simulink model "VTOL_sim_f_no_zeros"  (R2016b)
settings: Solver=ode45  StartTime=0.0  StopTime=200  RelTol=1e-3  EnableMultiTasking=on
InitFcn:
  | addpath ./..
  | VTOL_param
  | VTOLParamHWf_longitudinal
  | VTOLParamHWf_lateral
values from neighbouring files (symbols this model uses):
  denCh = [1/0.8 1]    [VTOLParamHWf_longitudinal.m]
  denth = [1/12 1]    [VTOLParamHWf_lateral.m]
  denz = [1/1 1]    [VTOLParamHWf_lateral.m]
  Kh = 0.066    [VTOLParamHWf_longitudinal.m]
  Kth = 0.31    [VTOLParamHWf_lateral.m]
  Kz = -0.006    [VTOLParamHWf_lateral.m]
  numCh = [1/0.14 1]    [VTOLParamHWf_longitudinal.m]
  numth = [1/1.6 1]    [VTOLParamHWf_lateral.m]
  numz = [1/0.18 1]    [VTOLParamHWf_lateral.m]
undefined symbols (not defined in the file or in its folder): P, VTOL_animation
settings Model: Creator=beard  LastModifiedBy=mclain
settings DataIOCC: LimitDataPoints=on  SaveFormat=Array  SignalLoggingSaveFormat=ModelDataLogs
settings OptimizationCC: ExpressionDepthLimit=2147483647  InitFltsAndDblsToZero=on  LifeSpan=inf
settings DebuggingCC: UnderspecifiedInitializationDetection=Classic  MergeDetectMultiDrivingBlocksExec=none  SolverPrmCheckMsg=warning  FcnCallInpInsideContextMsg=warning  StateNameClashWarn=warning  SFUnexpectedBacktrackingDiag=warning  SFNoUnconditionalDefaultTransitionDiag=warning  SFExecutionAtInitializationDiag=none
settings HardwareCC: ProdBitPerPointer=32  ProdBitPerSizeT=32  ProdBitPerPtrDiffT=32  ProdLargestAtomicFloat=None  ProdIntDivRoundTo=Undefined  ProdEndianess=Unspecified  ProdWordSize=32  ProdHWDeviceType=32-bit Generic
settings ModelReferenceCC: PropagateSignalLabelsOutOfModel=off
settings GRTTargetCC: TargetLangStandard=C89/C90 (ANSI)  GeneratePreprocessorConditionals=Disable all  CombineOutputUpdateFcns=off  GRTInterface=on
settings ConfigComp: CovMetricSettings=dw  CovHtmlReporting=on  CovSaveCumulativeToWorkspaceVar=on  CovSaveSingleToWorkspaceVar=on  CovExternalEMLEnable=off

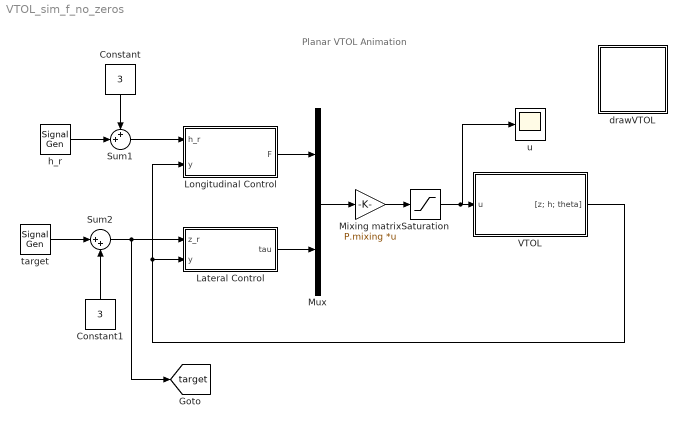
== system VTOL_sim_f_no_zeros ==
  note: Planar VTOL Animation
  Constant : Constant  Value=3
  Constant1 : Constant  Value=3
  Lateral Control : Subsystem
  Longitudinal Control : Subsystem
  Mixing matrix : Gain  Gain=P.mixing  Multiplication=Matrix(K*u)
  Mux : Mux  Inputs=2
  Saturation : Saturate  UpperLimit=100  LowerLimit=0
  Sum1 : Sum  Inputs=++|
  Sum2 : Sum  Inputs=|++
  VTOL : Subsystem
  drawVTOL : Subsystem
      mask Display: image(imread('tv.jpg'))
  h_r : SignalGenerator  WaveForm=square  Amplitude=2.5  Frequency=.01
  target : SignalGenerator  WaveForm=square  Amplitude=2  Frequency=.015
  u : Scope
  tag scope: target=global
  wires:
  VTOL/1("[z; h; theta]") -> Longitudinal Control/2(y), Lateral Control/2(y)
  Mux/1 -> Mixing matrix/1
  Mixing matrix/1 -> Saturation/1
  Longitudinal Control/1(F) -> Mux/1
  Lateral Control/1(tau) -> Mux/2
  Constant/1 -> Sum1/1
  Sum1/1 -> Longitudinal Control/1(h_r)
  h_r/1 -> Sum1/2
  target/1 -> Sum2/1
  Constant1/1 -> Sum2/2
  Saturation/1 -> u/1, VTOL/1(u)
  Sum2/1 -> [target], Lateral Control/1(z_r)

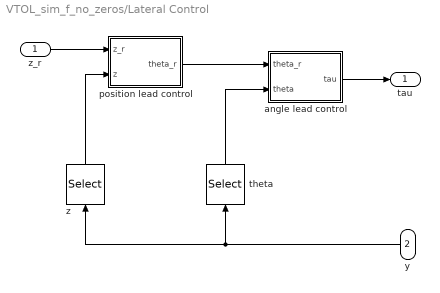
== system VTOL_sim_f_no_zeros/Lateral Control ==
  z_r : Inport
  y : Inport  Port=2
  "angle lead control " : Subsystem
  position lead control : Subsystem
  theta : Selector  InputPortWidth=3  IndexOptions=Index vector (dialog)  Indices=[3]  OutputSizes=1
  z : Selector  InputPortWidth=3  IndexOptions=Index vector (dialog)  Indices=[1]  OutputSizes=1
  tau : Outport
  wires:
  y/1 -> z/1, theta/1
  position lead control/1(theta_r) -> "angle lead control "/1(theta_r)
  theta/1 -> "angle lead control "/2(theta)
  z_r/1 -> position lead control/1(z_r)
  z/1 -> position lead control/2(z)
  "angle lead control "/1(tau) -> tau/1

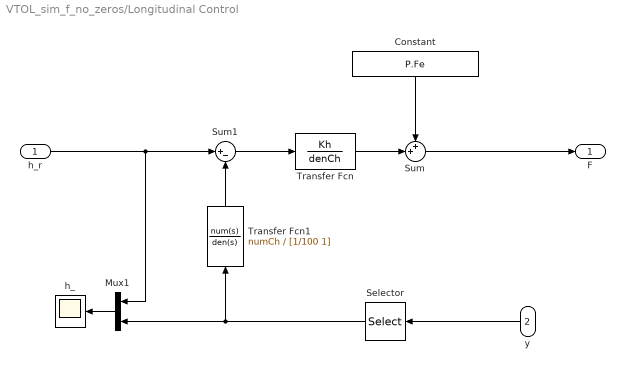
== system VTOL_sim_f_no_zeros/Longitudinal Control ==
  h_r : Inport
  y : Inport  Port=2
  Constant : Constant  Value=P.Fe
  Mux1 : Mux  Inputs=2
  Selector : Selector  InputPortWidth=3  IndexOptions=Index vector (dialog)  Indices=[2]  OutputSizes=1
  Sum : Sum  Inputs=++|
  Sum1 : Sum  Inputs=|+-
  Transfer Fcn : TransferFcn  Numerator=Kh  Denominator=denCh
  Transfer Fcn1 : TransferFcn  Numerator=numCh  Denominator=[1/100 1]
  h_ : Scope
  F : Outport
  wires:
  Selector/1 -> Transfer Fcn1/1, Mux1/2
  Sum/1 -> F/1
  Mux1/1 -> h_/1
  Constant/1 -> Sum/1
  h_r/1 -> Sum1/1, Mux1/1
  Sum1/1 -> Transfer Fcn/1
  y/1 -> Selector/1
  Transfer Fcn/1 -> Sum/2
  Transfer Fcn1/1 -> Sum1/2

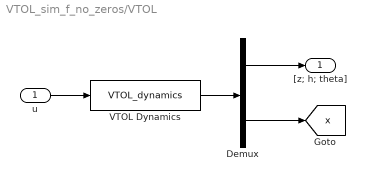
== system VTOL_sim_f_no_zeros/VTOL ==
  u : Inport
  Demux : Demux  Outputs=[3;6]
  VTOL Dynamics : S-Function  FunctionName=VTOL_dynamics  Parameters=P  SFunctionDeploymentMode=off  EnableBusSupport=off
  "[z; h; theta]" : Outport
  tag scope: x=global
  wires:
  u/1 -> VTOL Dynamics/1
  VTOL Dynamics/1 -> Demux/1
  Demux/1 -> "[z; h; theta]"/1
  Demux/2 -> [x]

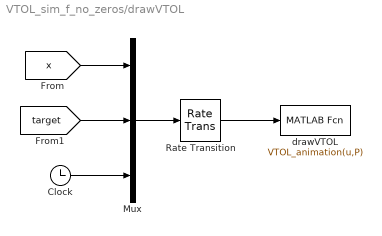
== system VTOL_sim_f_no_zeros/drawVTOL ==
  Clock : Clock
  Mux : Mux  Inputs=3
  Rate Transition : RateTransition  OutPortSampleTime=P.t_plot
  drawVTOL : MATLABFcn  MATLABFcn=VTOL_animation(u,P)  OutputDimensions=0
  wires:
  Mux/1 -> Rate Transition/1
  [x] -> Mux/1
  Clock/1 -> Mux/3
  Rate Transition/1 -> drawVTOL/1
  [target] -> Mux/2

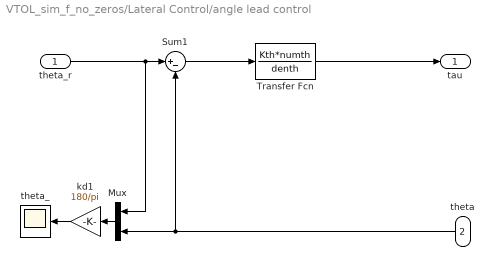
== system VTOL_sim_f_no_zeros/Lateral Control/angle lead control  ==
  theta_r : Inport
  theta : Inport  Port=2
  Mux : Mux  Inputs=2
  Sum1 : Sum  Inputs=|+-
  Transfer Fcn : TransferFcn  Numerator=Kth*numth  Denominator=denth
  kd1 : Gain  Gain=180/pi
  theta_ : Scope
  tau : Outport
  wires:
  theta_r/1 -> Sum1/1, Mux/1
  theta/1 -> Sum1/2, Mux/2
  Sum1/1 -> Transfer Fcn/1
  kd1/1 -> theta_/1
  Mux/1 -> kd1/1
  Transfer Fcn/1 -> tau/1

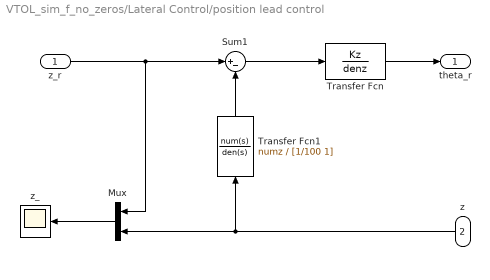
== system VTOL_sim_f_no_zeros/Lateral Control/position lead control ==
  z_r : Inport
  z : Inport  Port=2
  Mux : Mux  Inputs=2
  Sum1 : Sum  Inputs=|+-
  Transfer Fcn : TransferFcn  Numerator=Kz  Denominator=denz
  Transfer Fcn1 : TransferFcn  Numerator=numz  Denominator=[1/100 1]
  z_ : Scope
  theta_r : Outport
  wires:
  z_r/1 -> Sum1/1, Mux/1
  z/1 -> Transfer Fcn1/1, Mux/2
  Mux/1 -> z_/1
  Sum1/1 -> Transfer Fcn/1
  Transfer Fcn/1 -> theta_r/1
  Transfer Fcn1/1 -> Sum1/2
